simulink model "Test1"  (R2023a)
settings: Solver=VariableStepAuto  StartTime=0.0  StopTime=10.0  RelTol=1e-3
settings Model: Creator=16708  LastModifiedBy=16708

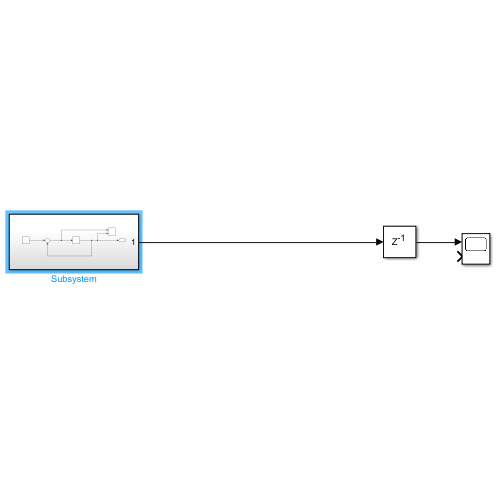
[thumbnail: Simulink's stored preview of the top-level diagram]
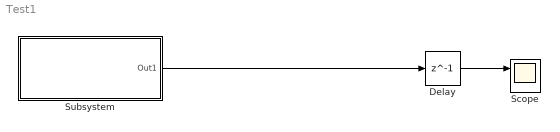
== system Test1 ==
  Delay : Delay  DelayLength=1  InitialCondition=0
  Scope : Scope  NumInputPorts=2
  Subsystem : Subsystem
  wires:
  Delay/1 -> Scope/1
  Subsystem/1(Out1) -> Delay/1

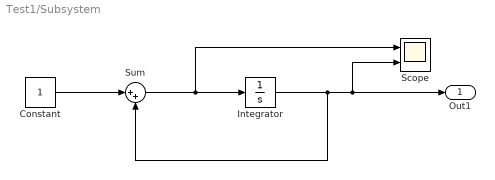
== system Test1/Subsystem ==
  Constant : Constant
  Integrator : Integrator
  Scope : Scope  NumInputPorts=2
  Sum : Sum  Inputs=|++
  Out1 : Outport
  wires:
  Sum/1 -> Scope/1, Integrator/1
  Constant/1 -> Sum/1
  Integrator/1 -> Scope/2, Out1/1, Sum/2
